simulink model "visualiser"  (R2022a)
settings: Solver=VariableStepAuto  StartTime=0.0  StopTime=Log.duration  RelTol=1e-3
InitFcn:
  | run('parameters.m')
  | run('initBusObjects.m')
settings Model: Creator=Chris  LastModifiedBy=chrismailer
settings ExplorerConfigSet: InternalSimMechanicsExplorerSettings="<ExplorerConfiguration><canonicalview>default</canonicalview><AnimationSetting><BasePlaybackSpeed>1.0</BasePlaybackSpeed><PlaybackSpeedFactor>0.125</PlaybackSpeedFactor></AnimationSetting><TilePanel><TileInfo><Tiles Columns=\"1\" Count=\"1\" Rows=\"1\"><Column Weight=\"1\"/><Row Weight=\"1\"/><Tile Height=\"1\" Width=\"1\" X=\"0\" Y=\"0\"/></Tiles></TileInfo><SceneInfo><SceneViewer><BGColor><R>1</R><G>1</G><B>1</B></BGColor><Camera><DoPerspective>on</DoPerspective><Position><X>0.613665576741074692</X><Y>-0.700000000000000289</Y><Z>-0.0982566750282758417</Z></Position><Center><X>0.616218696236923269</X><Y>-4.44089209850062616e-16</Y><Z>0.171731253555281183</Z></Center><Up><X>0</X><Y>0</Y><Z>1</Z></Up><ViewLimDist>1</ViewLimDist><YLim>0.466307658154998583</YLim><XLim>0.720391789216490497</XLim></Camera></SceneViewer></SceneInfo></TilePanel><MechEditorPanel><Cameras><Camera><Id>Camera1</Id><Value><Name>Camera</Name><NativeCamera><PositionTrackingFeature>Subsystem_Reference.Camera_Origin.R</PositionTrackingFeature><CenterTrackingFeature>Subsystem_Reference.Body_Mesh.R</CenterTrackingFeature><UpVectorTrackingFeature>Subsystem_Reference.World_Frame.W</UpVectorTrackingFeature><CenterTrackingOrigin>on</CenterTrackingOrigin><UpVectorTrackingDirection>+Z</UpVectorTrackingDirection></NativeCamera></Value></Camera></Cameras><GfxPanelCameraMap><MapElement CameraMLId=\"Camera1\" GfxPanelIndex=\"0\"/></GfxPanelCameraMap><VideoCreator><PlaybackSpeedRatio>1.0</PlaybackSpeedRatio><FrameRate>60</FrameRate><VideoFormat>MPEG-4</VideoFormat><FrameSize>[1280 720]</FrameSize></VideoCreator></MechEditorPanel></ExplorerConfiguration>"

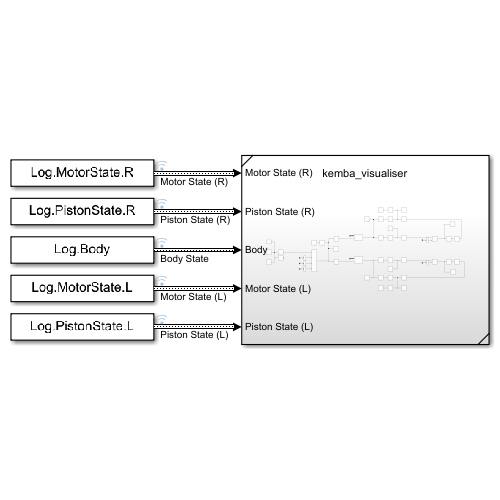
[thumbnail: Simulink's stored preview of the top-level diagram]
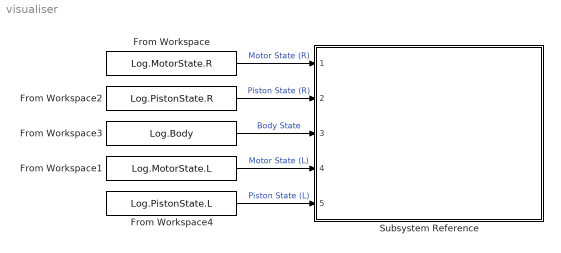
== system visualiser ==
  From Workspace : FromWorkspace  VariableName=Log.MotorState.R  OutDataTypeStr=Bus: MotorState  SampleTime=0.001  ZeroCross=off
  From Workspace1 : FromWorkspace  VariableName=Log.MotorState.L  OutDataTypeStr=Bus: MotorState  SampleTime=0.001
  From Workspace2 : FromWorkspace  VariableName=Log.PistonState.R  OutDataTypeStr=Bus: PistonState  SampleTime=0.001
  From Workspace3 : FromWorkspace  VariableName=Log.Body  OutDataTypeStr=Bus: BodyState  SampleTime=0.001
  From Workspace4 : FromWorkspace  VariableName=Log.PistonState.L  OutDataTypeStr=Bus: PistonState  SampleTime=0.001
  Subsystem Reference : Subsystem  ReferencedSubsystem=kemba_visualiser
  wires:
  From Workspace/1 -> Subsystem Reference/1  "Motor State (R)"
  From Workspace1/1 -> Subsystem Reference/4  "Motor State (L)"
  From Workspace2/1 -> Subsystem Reference/2  "Piston State (R)"
  From Workspace3/1 -> Subsystem Reference/3  "Body State"
  From Workspace4/1 -> Subsystem Reference/5  "Piston State (L)"
